simulink model "Assignment2_V2_5_FINAL_INTEGRATION"  (R2017b)
settings: Solver=FixedStepAuto  StartTime=0.0  StopTime=inf  FixedStep=0.001  RelTol=1e-3  EnableMultiTasking=on
undefined symbols (not defined in the file): A0, A1, D0, D1, D10, D11, D12, D13, D2, D3, D5, D6, D8, D9, PTA0, PTA1, PTA2, PTB2, PTB3, PTB9, PTC16, PTC17, PTC2, PTC4, PTD0, PTD1, PTD2, PTD3
libraries: frdmk64flib x30, etargetslib x1
settings Model: ExtModeTrigDuration=5  Creator=montema2  LastModifiedBy=farona
settings OptimizationCC: PassReuseOutputArgsAs=Individual arguments  MaxStackSize=64
settings DebuggingCC: ParameterTunabilityLossMsg=error
settings HardwareCC: ProdBitPerPointer=32  ProdBitPerSizeT=32  ProdBitPerPtrDiffT=32  ProdLargestAtomicInteger=Long  ProdLargestAtomicFloat=Double  ProdWordSize=32  ProdHWDeviceType=ARM Compatible->ARM Cortex
settings SFSimCC: MATLABDynamicMemAlloc=off
settings RTWCC: SystemTargetFile=ert.tlc  HardwareBoard=NXP FRDM-K64F  TemplateMakefile=ert_default_tmf  GenerateReport=on  Toolchain=GNU Tools for ARM Embedded Processors  IncludeHyperlinkInReport=on  LaunchReport=on  GenerateTraceInfo=on  GenerateTraceReport=on  GenerateTraceReportSl=on  GenerateTraceReportSf=on  GenerateTraceReportEml=on
settings CodeAppCC: ForceParamTrailComments=on  IgnoreCustomStorageClasses=off  OperatorAnnotations=on  SimulinkDataObjDesc=on  SFDataObjDesc=on  InsertBlockDesc=on

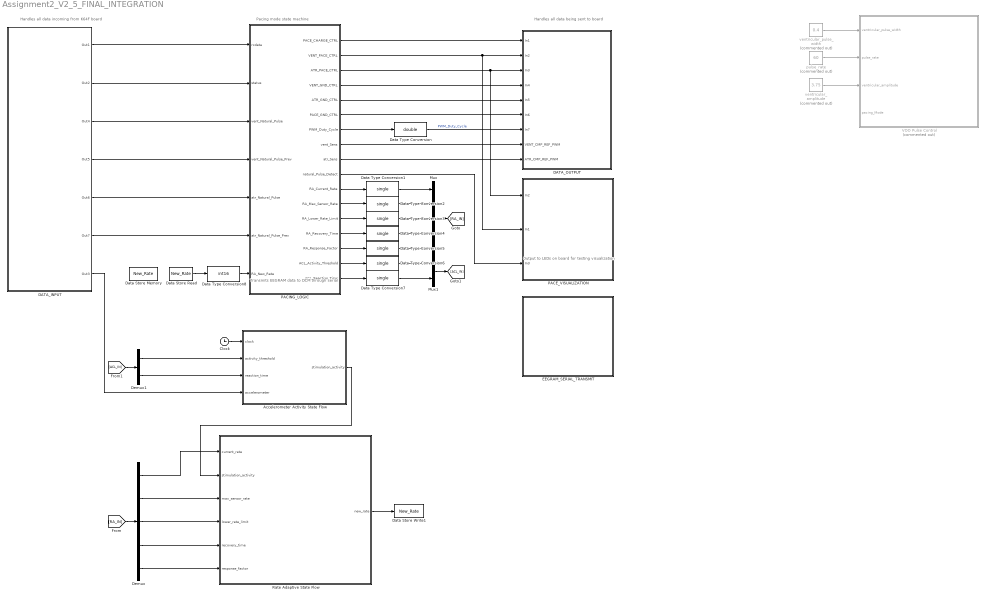
== system Assignment2_V2_5_FINAL_INTEGRATION ==
  note: Output to LEDs on board for testing visualization
  note: Transmits EEGRAM data to DCM through serial
  note: Handles all data being sent to board
  note: Handles all data incoming from K64F board
  note: Pacing mode state machine
  "Accelerometer Activity State Flow " : Stateflow chart  TreatAsAtomicUnit=on
  Clock : Clock
  DATA_INPUT : Subsystem
  DATA_OUTPUT : Subsystem
  Data Store Memory : DataStoreMemory  DataStoreName=New_Rate  ReadBeforeWriteMsg=warning  WriteAfterWriteMsg=warning  WriteAfterReadMsg=warning  InitialValue=60  ShowAdditionalParam=off  OutDataTypeStr=single
  Data Store Read : DataStoreRead  DataStoreName=New_Rate  DataStoreElements=New_Rate
  Data Store Write1 : DataStoreWrite  DataStoreName=New_Rate  DataStoreElements=New_Rate
  Data Type Conversion : DataTypeConversion  OutDataTypeStr=double  RndMeth=Nearest
  Data Type Conversion{1..7} (7 alike) : DataTypeConversion  OutDataTypeStr=single  RndMeth=Nearest
  Data Type Conversion8 : DataTypeConversion  OutDataTypeStr=int16  RndMeth=Nearest
  Demux : Demux  Outputs=5
  Demux1 : Demux  Outputs=2
  EEGRAM_SERIAL_TRANSMIT : Subsystem
  Mux : Mux  Inputs=5
  Mux1 : Mux  Inputs=2
  PACE_VISUALIZATION : Subsystem
  PACING_LOGIC : Stateflow chart  TreatAsAtomicUnit=on
  "Rate Adaptive State Flow " : Stateflow chart  TreatAsAtomicUnit=on
  VOO Pulse Control : Subsystem  Commented=on
  pulse_rate : Constant  Commented=on  Value=60  OutMin=[50]  OutMax=[175]
  ventricular_amplitude : Constant  Commented=on  Value=3.75
  ventricular_pulse_width : Constant  Commented=on  Value=0.4
  wires:
  ventricular_pulse_width/1 -> VOO Pulse Control/1(ventricular_pulse_width)
  pulse_rate/1 -> VOO Pulse Control/2(pulse_rate)
  ventricular_amplitude/1 -> VOO Pulse Control/3(ventricular_amplitude)
  PACING_LOGIC/4(VENT_GND_CTRL) -> DATA_OUTPUT/4(In4)
  PACING_LOGIC/6(PACE_GND_CTRL) -> DATA_OUTPUT/6(In6)
  PACING_LOGIC/1(PACE_CHARGE_CTRL) -> DATA_OUTPUT/1(In1)
  PACING_LOGIC/7(PWM_Duty_Cycle) -> Data Type Conversion/1
  PACING_LOGIC/5(ATR_GND_CTRL) -> DATA_OUTPUT/5(In5)
  PACING_LOGIC/2(VENT_PACE_CTRL) -> PACE_VISUALIZATION/2(In1), DATA_OUTPUT/2(In2)
  PACING_LOGIC/3(ATR_PACE_CTRL) -> PACE_VISUALIZATION/1(In2), DATA_OUTPUT/3(In3)
  PACING_LOGIC/10(natural_Pulse_Detect) -> PACE_VISUALIZATION/3(In3)
  Data Type Conversion/1 -> DATA_OUTPUT/7(In7)  "PWM_Duty_Cycle"
  DATA_INPUT/1(Out1) -> PACING_LOGIC/1(rxdata)
  DATA_INPUT/2(Out2) -> PACING_LOGIC/2(status)
  DATA_INPUT/7(Out3) -> "Accelerometer Activity State Flow "/4(accelerometer)
  DATA_INPUT/3(Out4) -> PACING_LOGIC/3(vent_Natural_Pulse)
  DATA_INPUT/4(Out5) -> PACING_LOGIC/4(vent_Natural_Pulse_Prev)
  DATA_INPUT/5(Out6) -> PACING_LOGIC/5(atr_Natural_Pulse)
  DATA_INPUT/6(Out7) -> PACING_LOGIC/6(atr_Natural_Pulse_Prev)
  PACING_LOGIC/8(vent_Sens) -> DATA_OUTPUT/8(VENT_CMP_REF_PWM)
  PACING_LOGIC/9(atr_Sens) -> DATA_OUTPUT/9(ATR_CMP_REF_PWM)
  Clock/1 -> "Accelerometer Activity State Flow "/1(clock)
  Data Store Read/1 -> Data Type Conversion8/1
  "Rate Adaptive State Flow "/1(new_rate) -> Data Store Write1/1
  Mux/1 -> [RA_IN]
  PACING_LOGIC/15(RA_Response_Factor) -> Data Type Conversion5/1
  PACING_LOGIC/14(RA_Recovery_Time) -> Data Type Conversion4/1
  PACING_LOGIC/13(RA_Lower_Rate_Limit) -> Data Type Conversion3/1
  PACING_LOGIC/12(RA_Max_Sensor_Rate) -> Data Type Conversion2/1
  PACING_LOGIC/11(RA_Current_Rate) -> Data Type Conversion1/1
  [RA_IN] -> Demux/1
  Demux/1 -> "Rate Adaptive State Flow "/1(current_rate)
  Demux/2 -> "Rate Adaptive State Flow "/3(max_sensor_rate)
  Demux/3 -> "Rate Adaptive State Flow "/4(lower_rate_limit)
  Demux/4 -> "Rate Adaptive State Flow "/5(recovery_time)
  Demux/5 -> "Rate Adaptive State Flow "/6(response_factor)
  "Accelerometer Activity State Flow "/1(stimulation_activity) -> "Rate Adaptive State Flow "/2(stimulation_activity)
  PACING_LOGIC/17(ACL_Reaction_Time) -> Data Type Conversion7/1
  PACING_LOGIC/16(ACL_Activity_Threshold) -> Data Type Conversion6/1
  Mux1/1 -> [ACL_IN]
  [ACL_IN] -> Demux1/1
  Demux1/1 -> "Accelerometer Activity State Flow "/2(activity_threshold)
  Demux1/2 -> "Accelerometer Activity State Flow "/3(reaction_time)
  Data Type Conversion1/1 -> Mux/1
  Data Type Conversion2/1 -> Mux/2
  Data Type Conversion3/1 -> Mux/3
  Data Type Conversion4/1 -> Mux/4
  Data Type Conversion5/1 -> Mux/5
  Data Type Conversion6/1 -> Mux1/1
  Data Type Conversion7/1 -> Mux1/2
  Data Type Conversion8/1 -> PACING_LOGIC/7(RA_New_Rate)

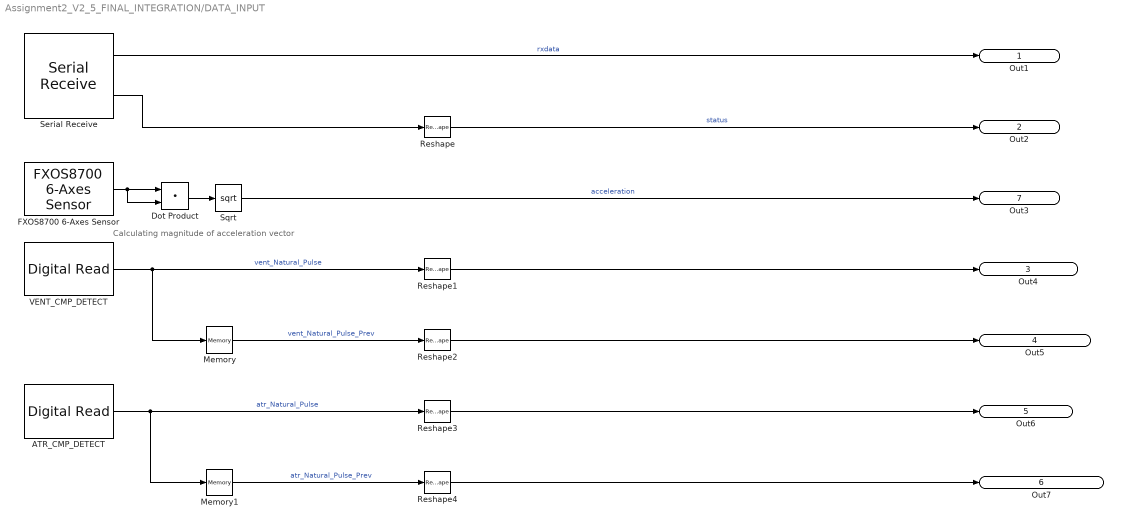
== system Assignment2_V2_5_FINAL_INTEGRATION/DATA_INPUT ==
  note: Calculating magnitude of acceleration vector
  ATR_CMP_DETECT : frdmk64flib/Digital Read  Whichpin=PTC16 (D0)  SampleTime=-1
      settings: SourceProductName=Simulink Coder Support Package for NXP FRDM-K64F Board
  Dot Product : DotProduct  InputSameDT=on  OutDataTypeStr=Inherit: Inherit via internal rule
  FXOS8700 6-Axes Sensor : frdmk64flib/FXOS8700 6-Axes Sensor  Activesensor=Accelerometer only  ODR=800Hz  HybridODR=400Hz  Accelfullrange=-2g to +2g  SampleTime=-1
      settings: SourceProductName=Simulink Coder Support Package for NXP FRDM-K64F Board
  Memory : Memory
  Memory1 : Memory
  Reshape{,1..4} (5 alike) : Reshape  OutputDimensionality=Customize  OutputDimensions=[1]
  Serial Receive : frdmk64flib/Serial Receive  SCIModule=0  Baudrate=uint32(9600)  Parity=None  StopBits=1  HardwareFlowControl=None  ByteOrder=LittleEndian  DataType=uint8  DataLength=44  BlockingMode=off  OutputStatus=on  SampleTime=-1
      settings: SourceProductName=Simulink Coder Support Package for NXP FRDM-K64F Board
  Sqrt : Sqrt  SaturateOnIntegerOverflow=on
  VENT_CMP_DETECT : frdmk64flib/Digital Read  Whichpin=PTC17 (D1)  SampleTime=-1
      settings: SourceProductName=Simulink Coder Support Package for NXP FRDM-K64F Board
  Out1 : Outport
  Out2 : Outport  Port=2
  Out4 : Outport  Port=3
  Out5 : Outport  Port=4
  Out6 : Outport  Port=5
  Out7 : Outport  Port=6
  Out3 : Outport  Port=7
  wires:
  Serial Receive/2 -> Reshape/1
  Serial Receive/1 -> Out1/1  "rxdata"
  Dot Product/1 -> Sqrt/1
  FXOS8700 6-Axes Sensor/1 -> Dot Product/2, Dot Product/1
  Reshape/1 -> Out2/1  "status"
  Sqrt/1 -> Out3/1  "acceleration"
  VENT_CMP_DETECT/1 -> Reshape1/1, Memory/1  "vent_Natural_Pulse"
  Memory/1 -> Reshape2/1  "vent_Natural_Pulse_Prev"
  Memory1/1 -> Reshape4/1  "atr_Natural_Pulse_Prev"
  ATR_CMP_DETECT/1 -> Reshape3/1, Memory1/1  "atr_Natural_Pulse"
  Reshape1/1 -> Out4/1
  Reshape2/1 -> Out5/1
  Reshape3/1 -> Out6/1
  Reshape4/1 -> Out7/1

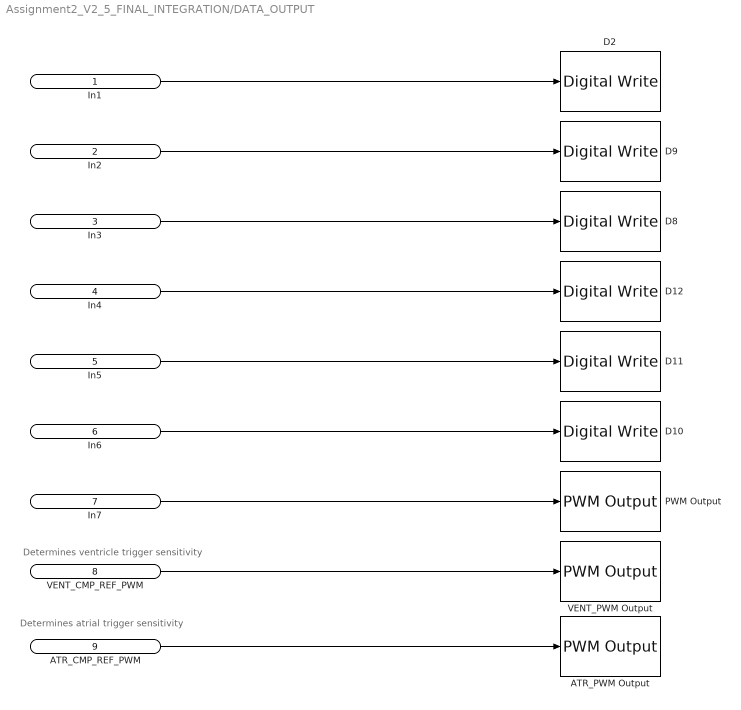
== system Assignment2_V2_5_FINAL_INTEGRATION/DATA_OUTPUT ==
  note: Determines ventricle trigger sensitivity
  note: Determines atrial trigger sensitivity
  In1 : Inport
  In2 : Inport  Port=2
  In3 : Inport  Port=3
  In4 : Inport  Port=4
  In5 : Inport  Port=5
  In6 : Inport  Port=6
  In7 : Inport  Port=7
  VENT_CMP_REF_PWM : Inport  Port=8
  ATR_CMP_REF_PWM : Inport  Port=9
  ATR_PWM Output : frdmk64flib/PWM Output  Whichpin=PTC2 (D6)  InitialFrequency=1000  InitialDutyCycle=0
      settings: SourceProductName=Simulink Coder Support Package for NXP FRDM-K64F Board
  D10 : frdmk64flib/Digital Write  Whichpin=PTD0 (D10)
      settings: SourceProductName=Simulink Coder Support Package for NXP FRDM-K64F Board
  D11 : frdmk64flib/Digital Write  Whichpin=PTD2 (D11)
      settings: SourceProductName=Simulink Coder Support Package for NXP FRDM-K64F Board
  D12 : frdmk64flib/Digital Write  Whichpin=PTD3 (D12)
      settings: SourceProductName=Simulink Coder Support Package for NXP FRDM-K64F Board
  D2 : frdmk64flib/Digital Write  Whichpin=PTB9 (D2)
      settings: SourceProductName=Simulink Coder Support Package for NXP FRDM-K64F Board
  D8 : frdmk64flib/Digital Write  Whichpin=PTA0 (D8)
      settings: SourceProductName=Simulink Coder Support Package for NXP FRDM-K64F Board
  D9 : frdmk64flib/Digital Write  Whichpin=PTC4 (D9)
      settings: SourceProductName=Simulink Coder Support Package for NXP FRDM-K64F Board
  PWM Output : frdmk64flib/PWM Output  Whichpin=PTA2 (D5)  InitialFrequency=1000  InitialDutyCycle=0
      settings: SourceProductName=Simulink Coder Support Package for NXP FRDM-K64F Board
  VENT_PWM Output : frdmk64flib/PWM Output  Whichpin=PTA1 (D3)  InitialFrequency=1000  InitialDutyCycle=0
      settings: SourceProductName=Simulink Coder Support Package for NXP FRDM-K64F Board
  wires:
  In1/1 -> D2/1
  In6/1 -> D10/1
  In2/1 -> D9/1
  In4/1 -> D12/1
  In3/1 -> D8/1
  In7/1 -> PWM Output/1
  In5/1 -> D11/1
  VENT_CMP_REF_PWM/1 -> VENT_PWM Output/1
  ATR_CMP_REF_PWM/1 -> ATR_PWM Output/1

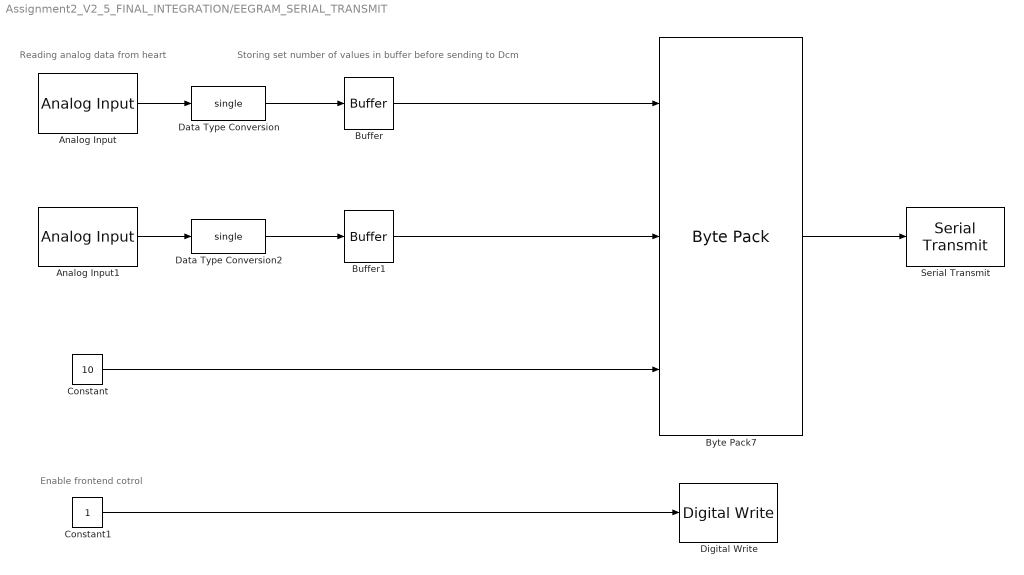
== system Assignment2_V2_5_FINAL_INTEGRATION/EEGRAM_SERIAL_TRANSMIT ==
  note: Enable frontend cotrol
  note: Storing set number of values in buffer before sending to Dcm
  note: Reading analog data from heart
  Analog Input : frdmk64flib/Analog Input  Whichpin=PTB2 (A0)  SampleTime=0.005
      settings: SourceProductName=Simulink Coder Support Package for NXP FRDM-K64F Board
  Analog Input1 : frdmk64flib/Analog Input  Whichpin=PTB3 (A1)  SampleTime=0.005
      settings: SourceProductName=Simulink Coder Support Package for NXP FRDM-K64F Board
  Buffer : Buffer  N=25  OutputFrames=off
  Buffer1 : Buffer  N=25  OutputFrames=off
  Byte Pack7 : etargetslib/Byte Pack  datatypes={'single', 'single', 'uint8'}  byteAlign=1
  Constant : Constant  Value=10  OutDataTypeStr=uint8
  Constant1 : Constant
  Data Type Conversion : DataTypeConversion  OutDataTypeStr=single
  Data Type Conversion2 : DataTypeConversion  OutDataTypeStr=single
  Digital Write : frdmk64flib/Digital Write  Whichpin=PTD1 (D13)
      settings: SourceProductName=Simulink Coder Support Package for NXP FRDM-K64F Board
  Serial Transmit : frdmk64flib/Serial Transmit  SCIModule=0  Baudrate=uint32(9600)  Parity=None  StopBits=1  HardwareFlowControl=None  ByteOrder=LittleEndian  BlockingMode=on  OutputStatus=off
      settings: SourceProductName=Simulink Coder Support Package for NXP FRDM-K64F Board
  wires:
  Byte Pack7/1 -> Serial Transmit/1
  Constant/1 -> Byte Pack7/3
  Analog Input/1 -> Data Type Conversion/1
  Analog Input1/1 -> Data Type Conversion2/1
  Data Type Conversion/1 -> Buffer/1
  Data Type Conversion2/1 -> Buffer1/1
  Buffer/1 -> Byte Pack7/1
  Buffer1/1 -> Byte Pack7/2
  Constant1/1 -> Digital Write/1

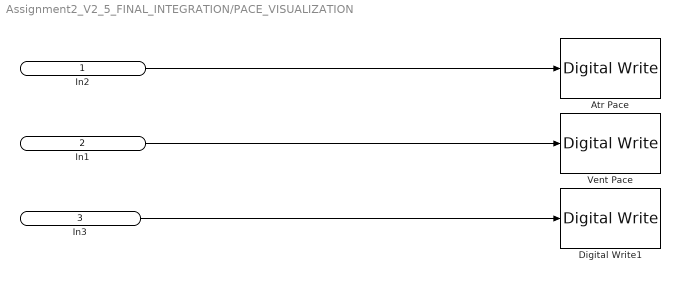
== system Assignment2_V2_5_FINAL_INTEGRATION/PACE_VISUALIZATION ==
  In2 : Inport
  In1 : Inport  Port=2
  In3 : Inport  Port=3
  Atr Pace : frdmk64flib/Digital Write  Whichpin=GREEN_LED
      settings: SourceProductName=Simulink Coder Support Package for NXP FRDM-K64F Board
  Digital Write1 : frdmk64flib/Digital Write  Whichpin=BLUE_LED
      settings: SourceProductName=Simulink Coder Support Package for NXP FRDM-K64F Board
  Vent Pace : frdmk64flib/Digital Write  Whichpin=RED_LED
      settings: SourceProductName=Simulink Coder Support Package for NXP FRDM-K64F Board
  wires:
  In3/1 -> Digital Write1/1
  In2/1 -> Atr Pace/1
  In1/1 -> Vent Pace/1

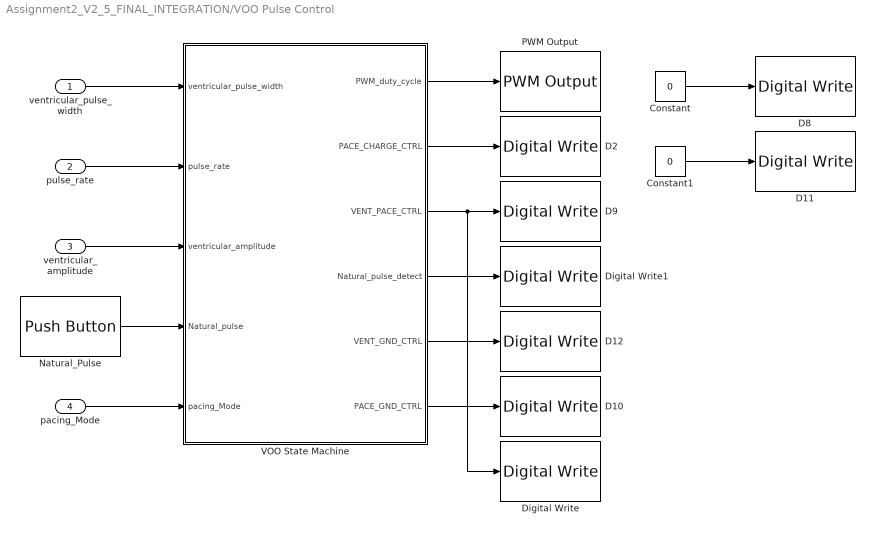
== system Assignment2_V2_5_FINAL_INTEGRATION/VOO Pulse Control ==
  ventricular_pulse_width : Inport
  pulse_rate : Inport  Port=2
  ventricular_amplitude : Inport  Port=3
  pacing_Mode : Inport  Port=4
  Constant : Constant  Value=0
  Constant1 : Constant  Value=0
  D10 : frdmk64flib/Digital Write  Whichpin=PTD0 (D10)
      settings: SourceProductName=Simulink Coder Support Package for NXP FRDM-K64F Board
  D11 : frdmk64flib/Digital Write  Whichpin=PTD2 (D11)
      settings: SourceProductName=Simulink Coder Support Package for NXP FRDM-K64F Board
  D12 : frdmk64flib/Digital Write  Whichpin=PTD3 (D12)
      settings: SourceProductName=Simulink Coder Support Package for NXP FRDM-K64F Board
  D2 : frdmk64flib/Digital Write  Whichpin=PTB9 (D2)
      settings: SourceProductName=Simulink Coder Support Package for NXP FRDM-K64F Board
  D8 : frdmk64flib/Digital Write  Whichpin=PTA0 (D8)
      settings: SourceProductName=Simulink Coder Support Package for NXP FRDM-K64F Board
  D9 : frdmk64flib/Digital Write  Whichpin=PTC4 (D9)
      settings: SourceProductName=Simulink Coder Support Package for NXP FRDM-K64F Board
  Digital Write : frdmk64flib/Digital Write  Whichpin=RED_LED
      settings: SourceProductName=Simulink Coder Support Package for NXP FRDM-K64F Board
  Digital Write1 : frdmk64flib/Digital Write  Whichpin=BLUE_LED
      settings: SourceProductName=Simulink Coder Support Package for NXP FRDM-K64F Board
  Natural_Pulse : frdmk64flib/Push Button  Whichswitch=SW2  SampleTime1=-1
      settings: SourceProductName=Simulink Coder Support Package for NXP FRDM-K64F Board
  PWM Output : frdmk64flib/PWM Output  Whichpin=PTA2 (D5)  InitialFrequency=1000  InitialDutyCycle=0
      settings: SourceProductName=Simulink Coder Support Package for NXP FRDM-K64F Board
  VOO State Machine : Stateflow chart  TreatAsAtomicUnit=on
  wires:
  ventricular_pulse_width/1 -> VOO State Machine/1(ventricular_pulse_width)
  VOO State Machine/1(PWM_duty_cycle) -> PWM Output/1
  VOO State Machine/3(VENT_PACE_CTRL) -> Digital Write/1, D9/1
  pulse_rate/1 -> VOO State Machine/2(pulse_rate)
  VOO State Machine/2(PACE_CHARGE_CTRL) -> D2/1
  VOO State Machine/5(VENT_GND_CTRL) -> D12/1
  VOO State Machine/6(PACE_GND_CTRL) -> D10/1
  Constant/1 -> D8/1
  Constant1/1 -> D11/1
  Natural_Pulse/1 -> VOO State Machine/4(Natural_pulse)
  VOO State Machine/4(Natural_pulse_detect) -> Digital Write1/1
  ventricular_amplitude/1 -> VOO State Machine/3(ventricular_amplitude)
  pacing_Mode/1 -> VOO State Machine/5(pacing_Mode)

== stateflow chart Assignment2_V2_5_FINAL_INTEGRATION/PACING_LOGIC ==
  note: VOO and VVI Pacing mode logic
  note: Discharge into heart
  note: Ventricle pacing initialization
  state VENT_CURRENT_IN
    entry:PWM_Duty_Cycle = vent_Pulse_Amp;
    PACE_CHARGE_CTRL=false;
    VENT_GND_CTRL=false;
    VENT_PACE_CTRL=true;
    RA_Current_Rate = RA_New_Rate;
  state VENTRICLE_INIT
    entry:VENT_PACE_CTRL=false;
    VENT_GND_CTRL=true;
    ATR_PACE_CTRL=false;
    ATR_GND_CTRL=true;
    PACE_CHARGE_CTRL=true;
    PACE_GND_CTRL=true;
  note: double check ATR_GND_CTRL state
  note: If in VVI mode this state is acccessible.
  note: Acts as standby mode if natural pace is detected.
  state INITIAL
    %Set intial values of parameters
    %VOO mode?
    entry: rateAdapt = 0;
    vent_Pulse_Width = 10; %milliseconds
    atr_Pulse_Width = 10;
    RA_Lower_Rate_Limit = 60; %bpm
    vent_Pulse_Amp = 3.5; %volts
    atr_Pulse_Amp = 3.5;
  state VENT_PULSE_SENSE
    entry: natural_Pulse_Detect = true;
    exit: natural_Pulse_Detect = false;
  state VENT_CURRENT_OUT
    entry:
    VENT_PACE_CTRL=false;
    PACE_CHARGE_CTRL=true;
    VENT_GND_CTRL=true;
    RA_Current_Rate = RA_New_Rate;
  note: Charge state
  state STANDBY
    %Wait for signal from DCM
  note: Serial recieve standby loop
  note: Check if pace mode is valid
  note: Checks if new signal has been received
      | from DCM. If so goes back to re-initialize
      | with new parameters.
  note: Parameter initialization with data received from DCM
  note: AOO and AAI pacing mode logic
  state PARAM_INIT
    entry: pace_Mode = typecast(rxdata(1:2), 'int16');
    RA_Lower_Rate_Limit = typecast(rxdata(3:4), 'int16');
    max_Rate_Lim = typecast(rxdata(5:6), 'int16');
    RA_Max_Sensor_Rate = typecast(rxdata(7:8), 'int16');
    fix_AV_Delay = typecast(rxdata(9:10), 'int16');
    vent_Pulse_Amp = (typecast(rxdata(11:14), 'single')/5)*100;
    atr_Pulse_Amp = (typecast(rxdata(15:18), 'single')/5)*100;
    vent_Pulse_Width = typecast(rxdata(19:20), 'int16');
    atr_Pulse_Width = typecast(rxdata(21:22), 'int16');
    vent_Sens = typecast(rxdata(23:26), 'single');
    atr_Sens = typecast(rxdata(27:30), 'single');
    VRP = typecast(rxdata(31:32), 'int16');
    ARP = typecast(rxdata(33:34), 'int16');
    PVARP = typecast(rxdata(35:36), 'int16');
    ACL_Activity_Threshold = typecast(rxdata(37:38), 'int16');
    ACL_Reaction_Time = typecast(rxdata(39:40), 'int16');
    RA_Response_Factor = typecast(rxdata(41:42), 'int16');
    RA_Recovery_Time = typecast(rxdata(43:44), 'int16');
    RA_Current_Rate = RA_Lower_Rate_Limit;
  note: Determine if mode is rate adaptive
  note: Goes to appropriate initialization state depending
      | on the mode passed from DCM. If data received is
      | invalid, returns to standby state to wait for next signal.
  note: Discharge into heart
  state PARAM_INIT_TEST [commented out]
    entry: pace_Mode = 5;
    min_Rate_Lim = 60;
    max_Rate_Lim = 120;
    max_Sensor_Rate = 100;
    fix_AV_Delay = 5; %msec
    vent_Pulse_Amp = (3.5/5)*100;
    atr_Pulse_Amp = (2.5/5)*100;
    vent_Pulse_Width = 10; %msec
    atr_Pulse_Width = 10; %msec
    vent_Sens = 80;
    atr_Sens = 80;
    VRP = 5; %msec
    ARP = 5; %msec
    PVARP = 5; %msec
    activity_Thresh = 1;
    reaction_Time = 3; %sec
    response_Factor = 8;
    recovery_Time = 120; %sec
  note: Atrial pacing initialization
  state ATR_CURRENT_IN
    entry:PWM_Duty_Cycle = atr_Pulse_Amp;
    PACE_CHARGE_CTRL=false;
    ATR_GND_CTRL=false;
    ATR_PACE_CTRL=true;
    RA_Current_Rate = RA_New_Rate;
  state SENS_CTRL
    state SENS_TRUE
      entry: SENSING = 1;
    state SENS_FALSE
      entry: SENSING = 0;
    SENS_TRUE -> (junction 191)
    (junction 187) -> SENS_TRUE [order 1] : [pace_Mode == 3 || pace_Mode == 4 || pace_Mode == 6 || pace_Mode == 9 || pace_Mode == 10 || pace_Mode == 12]
    (junction 187) -> SENS_FALSE [order 2]
    SENS_FALSE -> (junction 191)
  state ATRIAL_INIT
    entry:VENT_PACE_CTRL=false;
    VENT_GND_CTRL=true;
    ATR_PACE_CTRL=false;
    ATR_GND_CTRL=true;
    PACE_CHARGE_CTRL=true;
    PACE_GND_CTRL=true;
  note: Checks if selected mode has
      | natural pace sensing
  note: double check VENT_GND_CTRL state
  note: DOO and DOOR Initialization
  state DUAL_INIT
    entry:VENT_PACE_CTRL=false;
    VENT_GND_CTRL=true;
    ATR_PACE_CTRL=false;
    ATR_GND_CTRL=true;
    PACE_CHARGE_CTRL=true;
    PACE_GND_CTRL=true;
  state DDD_INIT
    %For assignment 3
  note: Charge state
  note: If in AAI mode this state is acccessible.
  state ATR_CURRENT_OUT
    entry:
    ATR_PACE_CTRL=false;
    PACE_CHARGE_CTRL=true;
    ATR_GND_CTRL=true;
    RA_Current_Rate = RA_New_Rate;
  note: Acts as standby mode if natural pace is detected.
  state ATR_PULSE_SENSE
    entry: natural_Pulse_Detect = true;
    exit: natural_Pulse_Detect = false;
  VENTRICLE_INIT -> VENT_CURRENT_IN [order 2] : [after((60000/RA_Current_Rate),msec)]
  (junction 191) -> (junction 7)
  (junction 328) -> VENTRICLE_INIT
  ATR_CURRENT_OUT -> VENT_CURRENT_IN [order 3] : [(pace_Mode ==  5 || pace_Mode ==11)&&(after((fix_AV_Delay),msec))]
  (junction 7) -> (junction 328) [order 1] : [pace_Mode ==1 || pace_Mode == 3 || pace_Mode ==7 || pace_Mode == 9]
  VENT_CURRENT_OUT -> VENT_CURRENT_IN [order 3] : [(pace_Mode == 1 || pace_Mode ==3 || pace_Mode == 7 || pace_Mode == 9)&&(after((60000/RA_Current_Rate)-(vent_Pulse_Width),msec))]
  VENT_CURRENT_IN -> VENT_CURRENT_OUT : [after((vent_Pulse_Width),msec)]
  VENTRICLE_INIT -> VENT_PULSE_SENSE [order 1] : [SENSING == 1 && vent_Natural_Pulse==true && vent_Natural_Pulse_Prev==false]
  (default) -> INITIAL
  VENT_PULSE_SENSE -> VENT_CURRENT_OUT
  VENT_CURRENT_OUT -> VENT_PULSE_SENSE [order 2] : [SENSING == 1 && vent_Natural_Pulse==true && vent_Natural_Pulse_Prev==false && after(VRP, msec)]
  INITIAL -> STANDBY
  VENT_CURRENT_OUT -> (junction 176) [order 1] : [status == 0]
  VENT_CURRENT_OUT -> ATR_CURRENT_IN [order 4] : [(pace_Mode ==  5 || pace_Mode ==11)&&(after((60000/RA_Current_Rate)-(vent_Pulse_Width)-(atr_Pulse_Width)-(fix_AV_Delay),msec))]
  (junction 7) -> STANDBY [order 5]
  (junction 5) -> STANDBY [order 2]
  STANDBY -> (junction 5) : [status == 0]
  (junction 176) -> (junction 5)
  (junction 5) -> (junction 38) [order 1] : [typecast(rxdata(1:2), 'int16') >= 0 && typecast(rxdata(1:2), 'int16') <= 12]
  ATR_CURRENT_OUT -> (junction 176) [order 1] : [status == 0]
  (junction 38) -> PARAM_INIT
  (junction 183) -> (junction 187)
  PARAM_INIT -> (junction 183) [order 1] : [pace_Mode <=5]{rateAdapt = 0}
  (junction 7) -> ATRIAL_INIT [order 2] : [pace_Mode ==2 || pace_Mode == 4 || pace_Mode ==8 || pace_Mode ==10]
  PARAM_INIT -> (junction 183) [order 2] : [pace_Mode > 6]{rateAdapt = 1}
  (junction 7) -> (junction 326) [order 3] : [pace_Mode ==5 || pace_Mode == 11]
  (junction 7) -> (junction 324) [order 4] : [pace_Mode ==6 || pace_Mode ==12 ]
  ATRIAL_INIT -> ATR_CURRENT_IN [order 2] : [after((60000/RA_Current_Rate),msec)]
  DUAL_INIT -> ATR_CURRENT_IN : [after((60000/RA_Current_Rate),msec)]
  DDD_INIT -> ATR_CURRENT_IN : [after((60000/RA_Current_Rate),msec)]
  ATR_CURRENT_OUT -> ATR_CURRENT_IN [order 2] : [(pace_Mode == 2 || pace_Mode == 4 || pace_Mode == 8 || pace_Mode == 10)&&(after((60000/RA_Current_Rate)-(atr_Pulse_Width),msec))]
  ATR_CURRENT_IN -> ATR_CURRENT_OUT : [after((atr_Pulse_Width),msec)]
  ATRIAL_INIT -> ATR_PULSE_SENSE [order 1] : [SENSING == 1 && atr_Natural_Pulse==true && atr_Natural_Pulse_Prev==false]
  (junction 326) -> DUAL_INIT
  (junction 324) -> DDD_INIT
  ATR_PULSE_SENSE -> ATR_CURRENT_OUT
  ATR_CURRENT_OUT -> ATR_PULSE_SENSE [order 4] : [SENSING == 1 && atr_Natural_Pulse==true && atr_Natural_Pulse_Prev==false && after(atr_Pulse_Width, msec)]
  data: rxdata input uint8; status input uint8; PACE_CHARGE_CTRL output boolean; VENT_PACE_CTRL output boolean; ATR_PACE_CTRL output boolean; VENT_GND_CTRL output boolean; ATR_GND_CTRL output boolean; PACE_GND_CTRL output boolean; PWM_Duty_Cycle output single; PVARP local int16; activity_Thresh local int16; max_Rate_Lim local int16; VRP local int16; ARP local int16; rateAdapt local; pace_Mode local int16; fix_AV_Delay local int16; atr_Pulse_Width local int16; vent_Pulse_Width local int16; vent_Pulse_Amp local single; atr_Pulse_Amp local single; vent_Natural_Pulse input boolean; vent_Natural_Pulse_Prev input boolean; atr_Natural_Pulse input boolean; atr_Natural_Pulse_Prev input boolean; vent_Sens output single; atr_Sens output single; natural_Pulse_Detect output; SENSING local int8; RA_Current_Rate output int16; RA_Max_Sensor_Rate output int16; RA_Lower_Rate_Limit output int16; RA_Recovery_Time output int16; RA_Response_Factor output int16; ACL_Activity_Threshold output int16; ACL_Reaction_Time output int16; RA_New_Rate input int16

== stateflow chart Assignment2_V2_5_FINAL_INTEGRATION/Accelerometer Activity State Flow  ==
  note: Accelerometer Activity State Flow
      | Takes input from the accelerometer as well as the DCM inputs for Activity Threshold and Reaction Time
      | and calculates whether the accelerometer data over one period of Reaction Time should be considered as
      | stimulation activity
  note: True State
      | True state immediatley returns to the counter state (while restarting the clock
      | and the counter) to check if stimulation activity should stay true
      | This state is entered if 2 or more samples record accelerometer activity
      | greater than the activity threshold.
  note: False State
      | Initialization state and false state sets stimulation activity
      | to false and resets the counter.
      | The only way to move out of this state is to detect
      | accelerometer activity greater than the activity threshold.
  state true_state
    entry:
    stimulation_activity = true;
    counter=0;
  state false_state
    entry:
    stimulation_activity = false;
    counter=0;
  note: Count State
      | Count state increments the counter which stores the number
      | of times acceleration activity has occured greater than activity
      | threshold within a reaction time cycle
      | This state occurs if accelerometer activity greater than the
      | activity threshold was detected, and it hasn't been a full
      | cycle of reaction time since the first activity
  note: No Count State
      | This state occurs if no accelerometer activity greater
      | than the activity threshold was detected, but it hasn't been
      | a full cycle of reaction time since the first activity (since
      | false or true state)
  state no_count_state
    entry:
    compare=clock-starttime;
  state count_state
    entry:
    counter=counter+1;
    compare=clock-starttime;
  note: No Count State and Count State sample the accelerometer data 20 times per reaction time cycle
  (default) -> false_state
  no_count_state -> false_state [order 3] : [compare>=reaction_time]
  count_state -> false_state [order 4] : [compare>=reaction_time]
  false_state -> count_state : [accelerometer >= activity_threshold]
      | {starttime=clock}
  true_state -> count_state : {starttime=clock}
  count_state -> true_state [order 1] : [counter>=2]
  no_count_state -> count_state [order 1] : [accelerometer >= activity_threshold && compare < reaction_time && after(reaction_time/20,sec)]
  count_state -> no_count_state [order 3] : [compare < reaction_time && after(reaction_time/20,sec)]
  no_count_state -> no_count_state [order 2] : [compare < reaction_time && after(reaction_time/20,sec)]
  count_state -> count_state [order 2] : [accelerometer >= activity_threshold && compare < reaction_time && after(reaction_time/20,sec)]
  data: clock input; stimulation_activity output boolean; activity_threshold input single; reaction_time input single; accelerometer input double; compare local; counter local int16; starttime local

== stateflow chart Assignment2_V2_5_FINAL_INTEGRATION/VOO Pulse Control/VOO State Machine ==
  note: Switch States:
      | true=closed
      | false=open
  state current_into_heart
    entry:
    PACE_CHARGE_CTRL=false;
    VENT_GND_CTRL=false;
    VENT_PACE_CTRL=true;
  state start_state
    entry:VENT_PACE_CTRL=false;
    VENT_GND_CTRL=true;
    PACE_CHARGE_CTRL=true;
    PACE_GND_CTRL=true;
    PWM_duty_cycle=((ventricular_amplitude/5)*100);
  state current_out_of_heart
    entry:
    VENT_PACE_CTRL=false;
    PACE_CHARGE_CTRL=true;
    VENT_GND_CTRL=true;
  state natural_pace
    entry: Natural_pulse_detect=true;
    exit: Natural_pulse_detect=false;
  (default) -> start_state
  start_state -> current_into_heart [order 1] : [after(((60/pulse_rate)*1000),msec)]
  current_into_heart -> natural_pace [order 2] : [Natural_pulse==true]
  start_state -> natural_pace [order 2] : [Natural_pulse==true]
  natural_pace -> start_state : [Natural_pulse==false]
  current_into_heart -> current_out_of_heart [order 1] : [after((ventricular_pulse_width),msec)]
  current_out_of_heart -> current_into_heart [order 1] : [after(((60/pulse_rate)*1000)-(ventricular_pulse_width),msec)]
  current_out_of_heart -> natural_pace [order 2] : [Natural_pulse==true]
  data: ventricular_pulse_width input double; pulse_rate input double; ventricular_amplitude input double; PWM_duty_cycle output double [0..100]; PACE_CHARGE_CTRL output boolean; VENT_PACE_CTRL output boolean; Natural_pulse_detect output; VENT_GND_CTRL output boolean; PACE_GND_CTRL output boolean; Natural_pulse input boolean; pacing_Mode input uint8

== stateflow chart Assignment2_V2_5_FINAL_INTEGRATION/Rate Adaptive State Flow  ==
  note: Rate Adaptive State Flow
      | This state flow controls the pacing rate depending on if stimulation activity was detected in the Accelerometer Activity State Flow.
      | In order to calculate the rate of increase and rate of decrease the DCM parameters for Maximum Sensor Rate, Lower Rate Limit, Recovery Time,
      | and Response Factor are needed.
      | This state flow outputs new_rate which is an updated rate used in the Pulsing State Flow. It takes, as input, current_rate which is the most
      | recently used rate in the Pulse State Flow.
  state initialization_state
    entry:
    posRoC = (max_sensor_rate/lower_rate_limit)*response_factor
    negRoC = (lower_rate_limit - max_sensor_rate)/(60*recovery_time)
  note: Initialization State
      | Calculates the positive and negative rates of change for the pace rate.
  note: Constant Lower Rate State
      | Maintains the output new_rate at the Lower Rate Limit
      | This state will only be returned to if the rate has decreased gradually
      | to the Lower Rate Limit on its own
  state const_lower_rate
    entry:new_rate = lower_rate_limit
  note: Increasing Rate State
      | If the stimulation activity becomes true and we have not
      | already reached the Maximum Sensor rate, this state is used.
      | Every second the new rate is calculated and updated if the newly
      | calculated rate will not go above the Maximum Sensor Rate
  note: Decreasing Rate State
      | If the stimulation activity ever becomes false, this state
      | is used. Every second the new rate is calculated and updated
      | if the newly calculated rate will not go below the Lower Rate Limit
  state increasing_rate
    entry:
    new_rate=current_rate + posRoC
  state decreasing_rate
    entry:
    new_rate=current_rate + negRoC
  state const_max_rate
    entry: new_rate=max_sensor_rate;
  note: Constant Max Rate State
      | If the rate has increased to the Maximum Sensor Rate this state is used.
      | Maintains the output new_rate at the Maximum Sensor Rate as long
      | as the stimulation activity stays true
  (default) -> initialization_state
  initialization_state -> const_lower_rate
  decreasing_rate -> const_lower_rate [order 2] : [after((1000),msec) && current_rate + negRoC <= lower_rate_limit]
  const_lower_rate -> increasing_rate : [stimulation_activity==true]
  increasing_rate -> decreasing_rate [order 1] : [stimulation_activity==false]
  increasing_rate -> increasing_rate [order 3] : [(current_rate + posRoC) < max_sensor_rate && after((1000),msec)]
  decreasing_rate -> decreasing_rate [order 3] : [after((1000),msec) && current_rate + negRoC > lower_rate_limit]
  decreasing_rate -> increasing_rate [order 1] : [stimulation_activity==true]
  increasing_rate -> const_max_rate [order 2] : [(current_rate + posRoC) >= max_sensor_rate && after((1000),msec)]
  const_max_rate -> decreasing_rate : [stimulation_activity==false]
  data: new_rate output single; current_rate input single; stimulation_activity input boolean; max_sensor_rate input single; lower_rate_limit input single; recovery_time input single; response_factor input single; posRoC local single; negRoC local single
